simulink model "three_phase_inverter_all_mode"  (R2019a)
settings: Solver=VariableStepAuto  StartTime=0.0  StopTime=.1  RelTol=1e-3
InitFcn:
  | clear all;
  | clc;
  | mode=180
  | freq=50
  | t=1/freq
  | pw=(mode/360)*100
libraries: powerlib x14
settings Model: Creator=Deepak  LastModifiedBy=Deepak

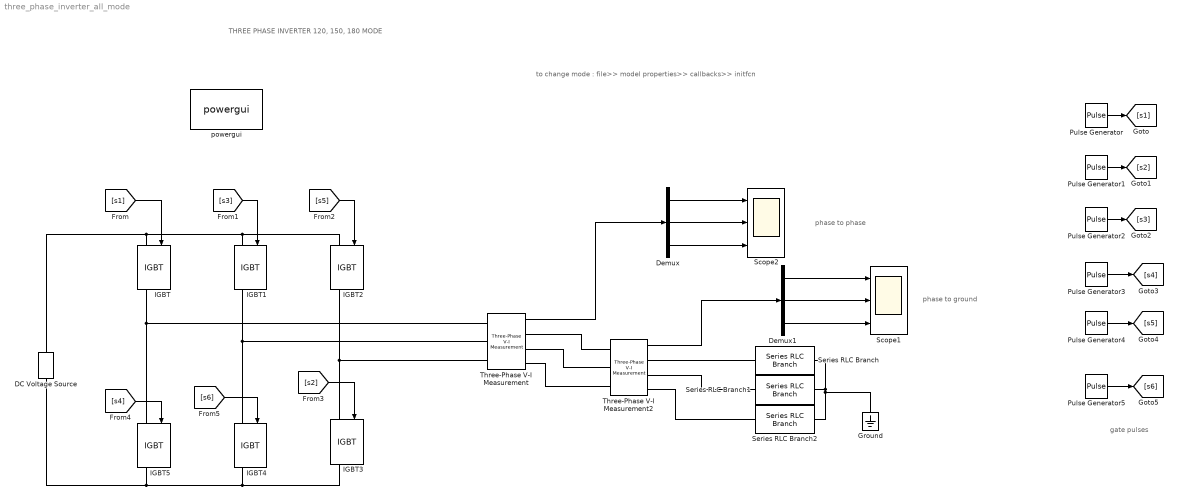
== system three_phase_inverter_all_mode ==
  note: gate pulses
  note: to change mode : file>> model properties>> callbacks>> initfcn
  note: phase to phase
  note: phase to ground
  note: THREE PHASE INVERTER 120, 150, 180 MODE
  DC Voltage Source : powerlib/Electrical Sources/DC Voltage Source  Amplitude=100  Measurements=None
      settings: SourceProductName=Simscape Electrical
  Demux : Demux  Outputs=3
  Demux1 : Demux  Outputs=3
  Ground : powerlib/Elements/Ground  LConnTagsString=a
      settings: SourceProductName=Simscape Electrical
  IGBT{,1..5} (6 alike) : powerlib/Power Electronics/IGBT  Ron=0.001  Lon=0  Vf=1  Tf=1e-6  Tt=2e-6  IC=0  Rs=1e5  Cs=inf  Measurements=on
      settings: SourceProductName=Simscape Electrical
  Pulse Generator : DiscretePulseGenerator  PulseType=Time based  Period=t  PulseWidth=pw
  Pulse Generator1 : DiscretePulseGenerator  PulseType=Time based  Period=t  PulseWidth=pw  PhaseDelay=t*(60/360)
  Pulse Generator2 : DiscretePulseGenerator  PulseType=Time based  Period=t  PulseWidth=pw  PhaseDelay=t*(120/360)
  Pulse Generator3 : DiscretePulseGenerator  PulseType=Time based  Period=t  PulseWidth=pw  PhaseDelay=t*(180/360)
  Pulse Generator4 : DiscretePulseGenerator  PulseType=Time based  Period=t  PulseWidth=pw  PhaseDelay=-t*(120/360)
  Pulse Generator5 : DiscretePulseGenerator  PulseType=Time based  Period=t  PulseWidth=pw  PhaseDelay=-t*(60/360)
  Scope1 : Scope  NumInputPorts=3
  Scope2 : Scope  NumInputPorts=3
  Series RLC Branch : powerlib/Elements/Series RLC Branch  LConnTagsString=__new0  RConnTagsString=__new0  BranchType=R  Resistance=10  Inductance=1e-3  SetiL0=off  InitialCurrent=0  Capacitance=1e-6  Setx0=off  InitialVoltage=0  Measurements=None
      settings: SourceProductName=Simscape Electrical
  Series RLC Branch1 : powerlib/Elements/Series RLC Branch  LConnTagsString=__new0  RConnTagsString=__new0  BranchType=R  Resistance=10  Inductance=1e-3  SetiL0=off  InitialCurrent=0  Capacitance=1e-6  Setx0=off  InitialVoltage=0  Measurements=None
      settings: SourceProductName=Simscape Electrical
  Series RLC Branch2 : powerlib/Elements/Series RLC Branch  LConnTagsString=__new0  RConnTagsString=__new0  BranchType=R  Resistance=10  Inductance=1e-3  SetiL0=off  InitialCurrent=0  Capacitance=1e-6  Setx0=off  InitialVoltage=0  Measurements=None
      settings: SourceProductName=Simscape Electrical
  Three-Phase V-I Measurement : powerlib/Measurements/Three-Phase V-I Measurement  VoltageMeasurement=phase-to-phase  SetLabelV=off  LabelV=Vabc  Vpu=off  VpuLL=off  CurrentMeasurement=no  SetLabelI=off  LabelI=Iabc  Ipu=off  Pbase=100e6  Vbase=500e3  OutputType=Complex  PhasorSimulation=off  PSBequivalent=0
      settings: SourceProductName=Simscape Electrical
  Three-Phase V-I Measurement2 : powerlib/Measurements/Three-Phase V-I Measurement  VoltageMeasurement=phase-to-ground  SetLabelV=off  LabelV=Vabc  Vpu=off  VpuLL=off  CurrentMeasurement=no  SetLabelI=off  LabelI=Iabc  Ipu=off  Pbase=100e6  Vbase=500e3  OutputType=Complex  PhasorSimulation=off  PSBequivalent=0
      settings: SourceProductName=Simscape Electrical
  powergui : powerlib/powergui  Priority=1  SimulationMode=Continuous  SampleTime=50e-6  frequency=60  Iterations=50  frequencyindice=0  Pbase=100e6  ErrMax=1e-4  UnitsV=kV  UnitsW=MW  buscounter=0  FunctionMessages=off  echomessages=off  EnableUseOfTLC=off  CurrentSourceSwitches=off  DisableSnubberDevices=off  DisableRonSwitches=off  DisableVfSwitches=off  DisplayEquations=off  AutomaticDiscreteSolvers=off  SolverType=Tustin/Backward Euler (TBE)  Interpol=off  ExternalGateDelay=off  methode=off  Ts=100  x0status=blocks  SPID=on  SwTol=0  HookPort=off  NonlinearTolerance=0  nMaxIteration=15  ContinueOnMaxIteration=off  RestoreLinks=warning  ResistiveCurrentMeasurement=off  Frange=[0:2:500]  Ylog=off  Xlog=on  ShowGrid=off  save=off  variable=ZData  structure=0  ZoomFFT=off  StartTime=0.0  cycles=1  DisplayStyle=1  fundamental=60  FreqAxis=off  MaxFrequency=1000  frequencyindicesteady=1  RmsSteady=1  display=off
      settings: SourceProductName=Simscape Electrical
  wires:
  [s1] -> IGBT/1
  [s6] -> IGBT4/1
  [s2] -> IGBT3/1
  [s4] -> IGBT5/1
  [s3] -> IGBT1/1
  [s5] -> IGBT2/1
  Pulse Generator3/1 -> [s4]
  Pulse Generator2/1 -> [s3]
  Pulse Generator4/1 -> [s5]
  Pulse Generator/1 -> [s1]
  Pulse Generator1/1 -> [s2]
  Pulse Generator5/1 -> [s6]
  Three-Phase V-I Measurement/1 -> Demux/1
  Three-Phase V-I Measurement2/1 -> Demux1/1
  Demux1/2 -> Scope1/2
  Demux1/1 -> Scope1/1
  Demux1/3 -> Scope1/3
  Demux/1 -> Scope2/1
  Demux/2 -> Scope2/2
  Demux/3 -> Scope2/3
  connections:
  IGBT2/RConn1 -- IGBT3/LConn1 -- Three-Phase V-I Measurement/LConn3
  IGBT1/RConn1 -- Three-Phase V-I Measurement/LConn2 -- IGBT4/LConn1
  IGBT/RConn1 -- IGBT5/LConn1 -- Three-Phase V-I Measurement/LConn1
  IGBT5/RConn1 -- IGBT4/RConn1 -- IGBT3/RConn1 -- DC Voltage Source/LConn1
  IGBT/LConn1 -- DC Voltage Source/RConn1 -- IGBT1/LConn1 -- IGBT2/LConn1
  Three-Phase V-I Measurement2/LConn1 -- Three-Phase V-I Measurement/RConn1
  Three-Phase V-I Measurement2/LConn2 -- Three-Phase V-I Measurement/RConn2
  Three-Phase V-I Measurement2/LConn3 -- Three-Phase V-I Measurement/RConn3
  Series RLC Branch/LConn1 -- Three-Phase V-I Measurement2/RConn1
  Series RLC Branch1/LConn1 -- Three-Phase V-I Measurement2/RConn2
  Series RLC Branch2/LConn1 -- Three-Phase V-I Measurement2/RConn3
  Series RLC Branch/RConn1 -- Series RLC Branch1/RConn1 -- Ground/LConn1 -- Series RLC Branch2/RConn1
